simulink model "x4Simulator"  (R2024b)
settings: Solver=ode3  StartTime=0.0  StopTime=60  FixedStep=0.0001  RelTol=1e-3
values from neighbouring files (symbols this model uses):
  alpha = 50    [run.m]
  c0 = zeros(3,mF)    [run.m]
  J = [2.098e3 63.577538 -2.002648 ... (first row only)    [run.m]
  k = 10    [run.m]
  Kd = diag([1 1 1])    [run.m]
  ki0 = 0.01*eye(3)    [run.m]
  m = 0.4    [run.m]
  rpy0 = [-pi/6 0.01 0.05]'    [run.m]
  s0 = compute_S(alpha,qt0,qtd0,w0,wd0)    [run.m]
  selected_control = 1    [run.m]
  w0 = [0 0 0]'    [run.m]
  wF = 10    [run.m]
  xi0 = [0 0 0]'    [run.m]
  xip0 = [0 0 0]'    [run.m]
  zd = 1    [run.m]
settings Model: Creator=ateverz  LastModifiedBy=ateveraz
settings OptimizationCC: ReuseModelBlockBuffer=off
settings RTWCC: GPUComputeCapability=3.5

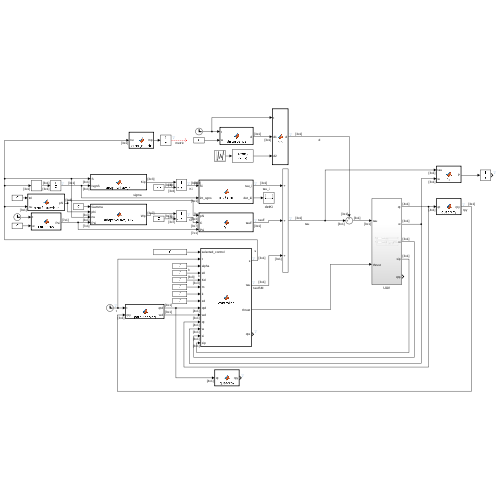
[thumbnail: Simulink's stored preview of the top-level diagram]
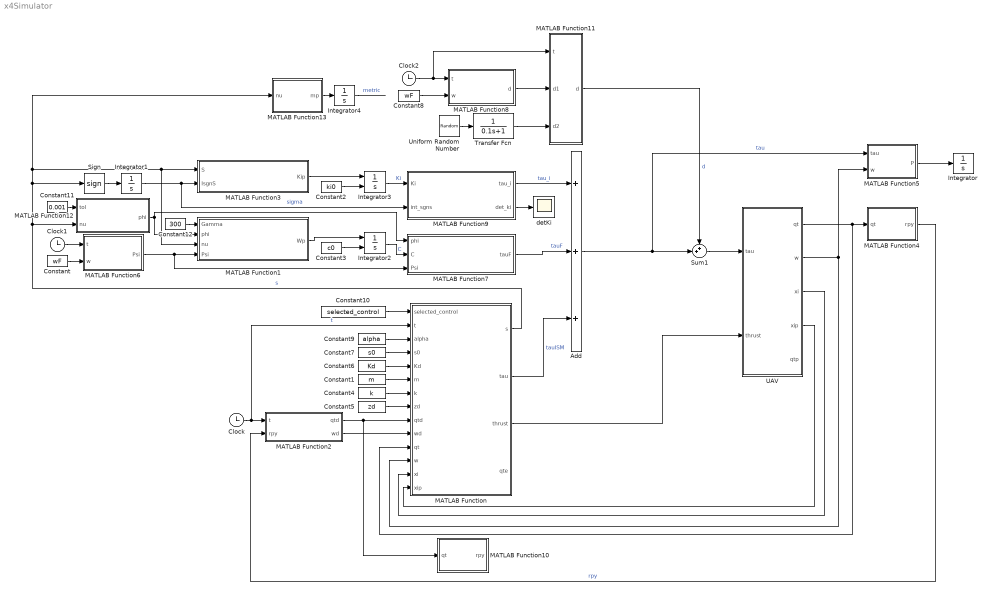
== system x4Simulator ==
  Add : Sum  Inputs=+++
  Clock : Clock
  Clock1 : Clock
  Clock2 : Clock
  Constant : Constant  Value=wF
  Constant1 : Constant  Value=m
  Constant10 : Constant  Value=selected_control
  Constant11 : Constant  Value=0.001
  Constant12 : Constant  Value=300
  Constant2 : Constant  Value=ki0
  Constant3 : Constant  Value=c0
  Constant4 : Constant  Value=k
  Constant5 : Constant  Value=zd
  Constant6 : Constant  Value=Kd
  Constant7 : Constant  Value=s0
  Constant8 : Constant  Value=wF
  Constant9 : Constant  Value=alpha
  Integrator : Integrator
  Integrator1 : Integrator  InitialCondition=[0 0 0]'
  Integrator2 : Integrator  InitialConditionSource=external  InitialCondition=c0
  Integrator3 : Integrator  InitialConditionSource=external  InitialCondition=zeros(3)
  Integrator4 : Integrator
  MATLAB Function : MATLAB Function  TreatAsAtomicUnit=on
  MATLAB Function1 : MATLAB Function  TreatAsAtomicUnit=on
  MATLAB Function10 : MATLAB Function  TreatAsAtomicUnit=on
  MATLAB Function11 : MATLAB Function  TreatAsAtomicUnit=on
  MATLAB Function12 : MATLAB Function  TreatAsAtomicUnit=on
  MATLAB Function13 : MATLAB Function  TreatAsAtomicUnit=on
  MATLAB Function2 : MATLAB Function  TreatAsAtomicUnit=on
  MATLAB Function3 : MATLAB Function  TreatAsAtomicUnit=on
  MATLAB Function4 : MATLAB Function  TreatAsAtomicUnit=on
  MATLAB Function5 : MATLAB Function  TreatAsAtomicUnit=on
  MATLAB Function6 : MATLAB Function  TreatAsAtomicUnit=on
  MATLAB Function7 : MATLAB Function  TreatAsAtomicUnit=on
  MATLAB Function8 : MATLAB Function  TreatAsAtomicUnit=on
  MATLAB Function9 : MATLAB Function  TreatAsAtomicUnit=on
  Sign : Signum
  Sum1 : Sum  Inputs=++|
  Transfer Fcn : TransferFcn  Denominator=[0.1 1]
  UAV : Subsystem
  Uniform Random Number : UniformRandomNumber  Minimum=-10  Maximum=10  SampleTime=.01
  detKi : Scope
  wires:
  Constant5/1 -> MATLAB Function/8(zd)
  Constant4/1 -> MATLAB Function/7(k)
  Constant1/1 -> MATLAB Function/6(m)
  UAV/2(w) -> MATLAB Function/12(w), MATLAB Function5/2(w)
  UAV/3(xi) -> MATLAB Function/13(xi)
  UAV/4(xip) -> MATLAB Function/14(xip)
  Constant6/1 -> MATLAB Function/5(Kd)
  UAV/1(qt) -> MATLAB Function/11(qt), MATLAB Function4/1(qt)
  Constant9/1 -> MATLAB Function/3(alpha)
  Clock/1 -> MATLAB Function2/1(t), MATLAB Function/2(t)  "t"
  MATLAB Function/3(thrust) -> UAV/2(thrust)
  MATLAB Function4/1(rpy) -> MATLAB Function2/2(rpy)  "rpy"
  MATLAB Function2/1(qtd) -> MATLAB Function10/1(qt), MATLAB Function/9(qtd)
  MATLAB Function2/2(wd) -> MATLAB Function/10(wd)
  MATLAB Function/1(s) -> MATLAB Function12/2(nu), MATLAB Function13/1(nu), MATLAB Function3/1(S), MATLAB Function1/3(nu), Sign/1  "s"
  Sign/1 -> Integrator1/1
  Integrator1/1 -> MATLAB Function9/2(int_sgns), MATLAB Function3/2(IsgnS)  "sigma"
  Clock1/1 -> MATLAB Function6/1(t)
  Constant/1 -> MATLAB Function6/2(w)
  MATLAB Function1/1(Wp) -> Integrator2/1
  MATLAB Function6/1(Psi) -> MATLAB Function7/3(Psi), MATLAB Function1/4(Psi)
  Integrator2/1 -> MATLAB Function7/2(C)  "C"
  MATLAB Function7/1(tauF) -> Add/2  "tauF"
  Constant3/1 -> Integrator2/2
  Clock2/1 -> MATLAB Function11/1(t), MATLAB Function8/1(t)
  Constant8/1 -> MATLAB Function8/2(w)
  MATLAB Function9/1(tau_i) -> Add/1  "tau_i"
  Integrator3/1 -> MATLAB Function9/1(Ki)  "Ki"
  MATLAB Function3/1(Kip) -> Integrator3/1
  Sum1/1 -> UAV/1(tau)
  MATLAB Function/2(tau) -> Add/3  "tauISM"
  Uniform Random Number/1 -> Transfer Fcn/1
  Constant2/1 -> Integrator3/2
  MATLAB Function8/1(d) -> MATLAB Function11/2(d1)
  Transfer Fcn/1 -> MATLAB Function11/3(d2)
  Add/1 -> MATLAB Function5/1(tau), Sum1/2  "tau"
  Constant7/1 -> MATLAB Function/4(s0)
  MATLAB Function5/1(P) -> Integrator/1
  MATLAB Function11/1(d) -> Sum1/1  "d"
  MATLAB Function9/2(det_ki) -> detKi/1
  Constant10/1 -> MATLAB Function/1(selected_control)
  Constant11/1 -> MATLAB Function12/1(tol)
  MATLAB Function12/1(phi) -> MATLAB Function1/2(phi), MATLAB Function7/1(phi)
  Constant12/1 -> MATLAB Function1/1(Gamma)
  MATLAB Function13/1(mp) -> Integrator4/1
  Integrator4/1 -> ?  "metric"

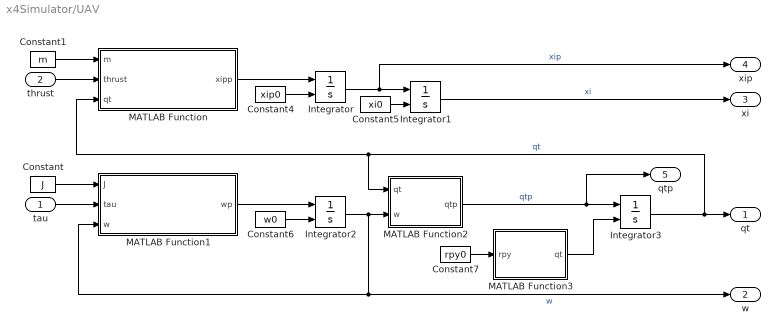
== system x4Simulator/UAV ==
  tau : Inport
  thrust : Inport  Port=2
  Constant : Constant  Value=J
  Constant1 : Constant  Value=m
  Constant4 : Constant  Value=xip0
  Constant5 : Constant  Value=xi0
  Constant6 : Constant  Value=w0
  Constant7 : Constant  Value=rpy0
  Integrator : Integrator  InitialConditionSource=external  InitialCondition=[0 0 0]'
  Integrator1 : Integrator  InitialConditionSource=external  InitialCondition=[0 0 0]'
  Integrator2 : Integrator  InitialConditionSource=external  InitialCondition=[0 0 0]'
  Integrator3 : Integrator  InitialConditionSource=external  InitialCondition=[0 0 0 0]'
  MATLAB Function : MATLAB Function  TreatAsAtomicUnit=on
  MATLAB Function1 : MATLAB Function  TreatAsAtomicUnit=on
  MATLAB Function2 : MATLAB Function  TreatAsAtomicUnit=on
  MATLAB Function3 : MATLAB Function  TreatAsAtomicUnit=on
  qt : Outport
  w : Outport  Port=2
  xi : Outport  Port=3
  xip : Outport  Port=4
  qtp : Outport  Port=5
  wires:
  Constant6/1 -> Integrator2/2
  Constant4/1 -> Integrator/2
  tau/1 -> MATLAB Function1/2(tau)
  Integrator2/1 -> MATLAB Function2/2(w), MATLAB Function1/3(w), w/1  "w"
  thrust/1 -> MATLAB Function/2(thrust)
  Integrator1/1 -> xi/1  "xi"
  Constant/1 -> MATLAB Function1/1(J)
  MATLAB Function3/1(qt) -> Integrator3/2
  MATLAB Function/1(xipp) -> Integrator/1
  MATLAB Function1/1(wp) -> Integrator2/1
  Constant7/1 -> MATLAB Function3/1(rpy)
  Integrator3/1 -> qt/1, MATLAB Function2/1(qt), MATLAB Function/3(qt)  "qt"
  Integrator/1 -> xip/1, Integrator1/1  "xip"
  Constant1/1 -> MATLAB Function/1(m)
  Constant5/1 -> Integrator1/2
  MATLAB Function2/1(qtp) -> qtp/1, Integrator3/1  "qtp"

== matlab function x4Simulator/MATLAB Function2 ==
  data: t input; qtd output; rpy input; wd output
function [qtd,wd] = pathPlanning(t,rpy)
        [qtd,wd] = reg1([0 0 0]); %tracking1(t,rpy);
end

== matlab function x4Simulator/MATLAB Function3 ==
  data: S input; Kip output; IsgnS input
function Kip = adaptiveLaw_Ki(S,IsgnS)
    Kip = adaptiveLaw_Ki(S,IsgnS);
end

== matlab function x4Simulator/MATLAB Function5 ==
  data: tau input; P output; w input
function P = fcn(tau, w)
    P = norm(tau'*w);
end

== matlab function x4Simulator/MATLAB Function6 ==
  data: t input; Psi output; w input
function Psi = FourierRV(t,w)
    mF = 7;
    Psi = FourierRV(t,w,mF);
end

== matlab function x4Simulator/MATLAB Function7 ==
  data: phi input; C input; tauF output; Psi input
function tauF = fcn(phi,C,Psi)
    tauF = - phi*C*Psi;
end

== matlab function x4Simulator/MATLAB Function8 ==
  data: t input; d output; w input
function d = disturbance(t,w)
    d = zeros(3,1);

    d(1) = cos(w*t) + sin(w*t);
    d(2) = - cos(w*t) + sin(w*t);
    d(3) = cos(w*t) - sin(w*t);
end

== matlab function x4Simulator/MATLAB Function9 ==
  data: Ki input; tau_i output; int_sgns input; det_ki output
function [tau_i, det_ki] = int_term(Ki,int_sgns)
    tau_i = - Ki*int_sgns;
    det_ki = det(Ki);
end

== matlab function x4Simulator/MATLAB Function10 ==
  data: qt input; rpy output
function rpy = quat2rpy(qt)
    rpy = quat2rpy(qt);
end

== matlab function x4Simulator/MATLAB Function11 ==
  data: t input; d output; d1 input; d2 input
function d = fcn(t,d1,d2)
    d  = zeros(3,1);
    if (t > 5 && t < 10 || t > 15 && t < 18 ||  t > 22 && t < 27) 
        d = d1 + d2;
    end
end

== matlab function x4Simulator/MATLAB Function12 ==
  data: tol input; nu input; phi output
function phi = errorSupervisor(tol, nu)
    phi = errorSupervisor(tol, nu);
end

== matlab function x4Simulator/MATLAB Function13 ==
  data: nu input; mp output
function mp = error_metric(nu)
    mp = nu'*nu;
end

== matlab function x4Simulator/UAV/MATLAB Function1 ==
  data: J input; wp output; tau input; w input
function wp = attitudeDynamics(J, tau, w)
    wp = attitudeDynamics(J, tau, w);
end

== matlab function x4Simulator/UAV/MATLAB Function ==
  data: m input; xipp output; thrust input; qt input
function xipp = cartesianDynamics(m, thrust, qt)
    xipp = cartesianDynamics(m, thrust, qt);
end

== matlab function x4Simulator/UAV/MATLAB Function2 ==
  data: qt input; w input; qtp output
function qtp = w2qtp(qt,w)
    qtp = w2qtp(qt,w);
end

== matlab function x4Simulator/UAV/MATLAB Function3 ==
  data: rpy input; qt output
function qt = rpy2quat(rpy)
    qt = rpy2quat(rpy);
end

== matlab function x4Simulator/MATLAB Function4 ==
  data: qt input; rpy output
function rpy = quat2rpy(qt)
    rpy = quat2rpy(qt);
end

== matlab function x4Simulator/MATLAB Function ==
  data: selected_control input; t input; s output; alpha input; s0 input; Kd input; tau output; m input; k input; zd input; qtd input; wd input; qt input; w input; xi input; xip input; thrust output; qte output
function [s, tau, thrust, qte] = controller(selected_control, t, alpha, s0, Kd, m, k, zd, qtd, wd,qt, w, xi, xip)
    if selected_control == 1    
        [tau, thrust, s, qte] = attitudeISMC(t, alpha, s0, Kd, m, k, zd, qtd, wd,qt, w, xi, xip);
    else
        [tau, thrust, s, qte] = ctrl_santibanez(t, alpha, s0, Kd, m, k, zd, qtd, wd,qt, w, xi, xip);
    end
end

== matlab function x4Simulator/MATLAB Function1 ==
  data: Gamma input; phi input; nu input; Wp output; Psi input
function Wp = adaptiveLaw_FNN(Gamma,phi, nu, Psi)
    Wp = adaptiveLaw_FNN(Gamma,phi, nu, Psi);
end
